simulink model "plot_atmos"  (Simulink 7.2)
settings: Solver=FixedStepDiscrete  StartTime=0.0  StopTime=10.0  FixedStep=dumTstep  RelTol=1e-3
libraries: auxvars_lib x2
settings Model: Creator=E183308  LastModifiedBy=E183308

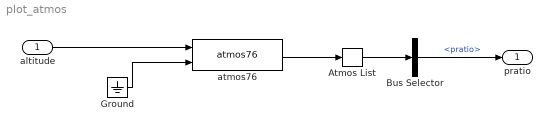
== system plot_atmos ==
  altitude : Inport  OutDataType=sfix(16)  OutScaling=2^0
  Atmos List : auxvars_lib/AuxiliaryVariables/Atmos76/Atmos List  SystemSampleTime=-1
  Bus Selector : BusSelector  OutputSignals=pratio
  Ground : Ground
  atmos76 : auxvars_lib/AuxiliaryVariables/Atmos76/atmos76  SystemSampleTime=-1
  pratio : Outport  OutDataType=sfix(16)  OutScaling=2^0
  wires:
  Ground/1 -> atmos76/2
  altitude/1 -> atmos76/1
  atmos76/1 -> Atmos List/1
  Atmos List/1 -> Bus Selector/1
  Bus Selector/1 -> pratio/1  "<pratio>"
